simulink model "wipercontrol"  (R2025a)
settings: Solver=FixedStepAuto  StartTime=0.0  StopTime=10.0  RelTol=1e-3
settings Model: DataDictionary=wiperData.sldd  Creator=nikul  LastModifiedBy=nikul
settings OptimizationCC: DefaultParameterBehavior=Inlined  EnhancedBackFolding=on  PassReuseOutputArgsAs=Individual arguments  ZeroExternalMemoryAtStartup=off  ZeroInternalMemoryAtStartup=off  OptimizeBlockOrder=speed  DifferentSizesBufferReuse=on  OptimizationCustomize=off  EfficientTunableParamExpr=on
settings DebuggingCC: ParameterTunabilityLossMsg=error
settings SFSimCC: MATLABDynamicMemAlloc=off
settings RTWCC: SystemTargetFile=ert.tlc  TemplateMakefile=ert_default_tmf  Description=Embedded Coder
settings CodeAppCC: ForceParamTrailComments=on  IgnoreCustomStorageClasses=off  OperatorAnnotations=on  SimulinkDataObjDesc=on  SFDataObjDesc=on  InsertBlockDesc=on
settings ERTTargetCC: ExtModeTransport=0.0  ExtModeStaticAlloc=off  ExtModeMexFile=ext_comm  ExtModeIntrfLevel=Level1  ERTCustomFileTemplate=example_file_process.tlc  TargetLangStandard=C99 (ISO)  GenerateSampleERTMain=on

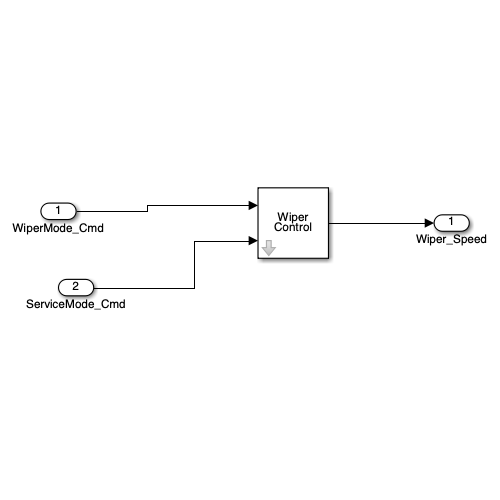
[thumbnail: Simulink's stored preview of the top-level diagram]
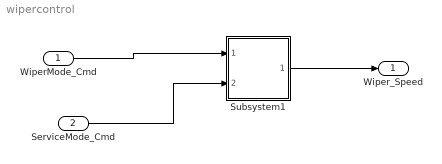
== system wipercontrol ==
  WiperMode_Cmd : Inport
  ServiceMode_Cmd : Inport  Port=2
  Subsystem1 : Subsystem  mask{WiperMode_Cmd=OFF|INTERMITTENT|LOW|HIGH, ServiceMode_Cmd=on}
      mask prompts: WiperMode_Cmd "Wiper Mode:"; ServiceMode_Cmd "Enable Service Mode"
      mask TypeOptions WiperMode_Cmd: OFF|INTERMITTENT|LOW|HIGH
      mask Display: disp('Wiper\nControl');
  Wiper_Speed : Outport
  wires:
  WiperMode_Cmd/1 -> Subsystem1/1(WiperMode_Cmd)
  ServiceMode_Cmd/1 -> Subsystem1/2(ServiceMode_Cmd)
  Subsystem1/1(Wiper_Speed) -> Wiper_Speed/1

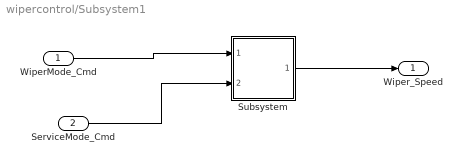
== system wipercontrol/Subsystem1 ==
  WiperMode_Cmd : Inport
  ServiceMode_Cmd : Inport  Port=2
  Subsystem : Subsystem
  Wiper_Speed : Outport
  wires:
  Subsystem/1(Wiper_Speed) -> Wiper_Speed/1
  ServiceMode_Cmd/1 -> Subsystem/2(ServiceMode_Cmd)
  WiperMode_Cmd/1 -> Subsystem/1(WiperMode_Cmd)

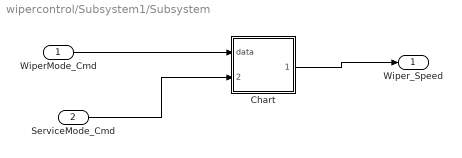
== system wipercontrol/Subsystem1/Subsystem ==
  WiperMode_Cmd : Inport
  ServiceMode_Cmd : Inport  Port=2
  Chart : Stateflow chart  TreatAsAtomicUnit=on
  Wiper_Speed : Outport
  wires:
  Chart/1(data2) -> Wiper_Speed/1
  WiperMode_Cmd/1 -> Chart/1(data)
  ServiceMode_Cmd/1 -> Chart/2(data1)

== stateflow chart wipercontrol/Subsystem1/Subsystem/Chart ==
  state ?
    state mode_high
      entry:
      Wiper_Speed = WiperSpeed_High;
    state normal
    state Service
    state Mode_intermittent
      state waiting
        entry :
        Wiper_Speed = 0;
        during:
        timer = timer+1;
      state wiping
        entry:
        Wiper_Speed = Wiper_Speed_low;
        timer = 0;
      wiping -> waiting : [after(1, sec)]
      (default) -> waiting
      waiting -> wiping : [timer >= Intermittent_Delay]
    state Mode_off
      entry:
      Wiper_Speed = 0;
    state mode_low
      entry:
      Wiper_Speed = WiperSpeed_Low;
    normal -> Service : [ServiceMode_Cmd == true]
    mode_high -> Mode_off : [WiperMode_cmd ~= WiperModes.HIGH]
    Mode_off -> mode_high [order 2] : [WiperMode_cmd == WiperModes.High]
    Service -> normal : [ServiceMode_Cmd == false]
    Mode_off -> Mode_intermittent [order 1] : [Wipermode_cmd == WiperModes.INTERMITTENT]
    (default) -> Mode_off
    Mode_off -> mode_low [order 3] : [WiperMode_cmd == WiperModes.Low]
    mode_low -> Mode_off : [WiperMode_Cmd ~= WiperModes.LOW]
    Mode_intermittent -> Mode_off : [WiperMode_Cmd ~= WiperModes.INTERMITTENT]
  data: timer local uint8; data input; data1 input; data2 output
